simulink model "Pod_elev_plant_mulecola"  (R2022b)
settings: Solver=VariableStepAuto  StartTime=0.0  StopTime=10.0  RelTol=1e-3
undefined symbols (not defined in the file): fix_conseg, fric_gear_elev, JLreg, JMreg, Kkeg, Kveg
settings Model: Creator=ohadformanair  LastModifiedBy=ohadformanair

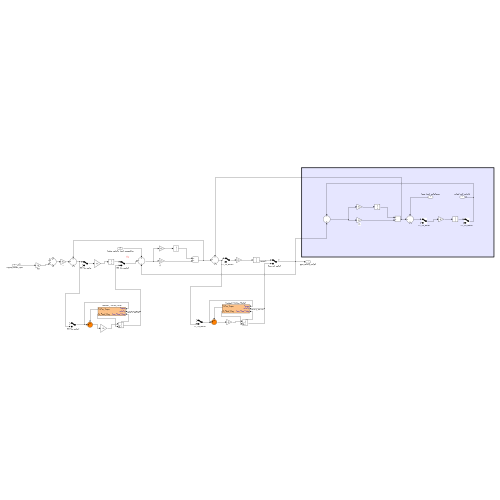
[thumbnail: Simulink's stored preview of the top-level diagram]
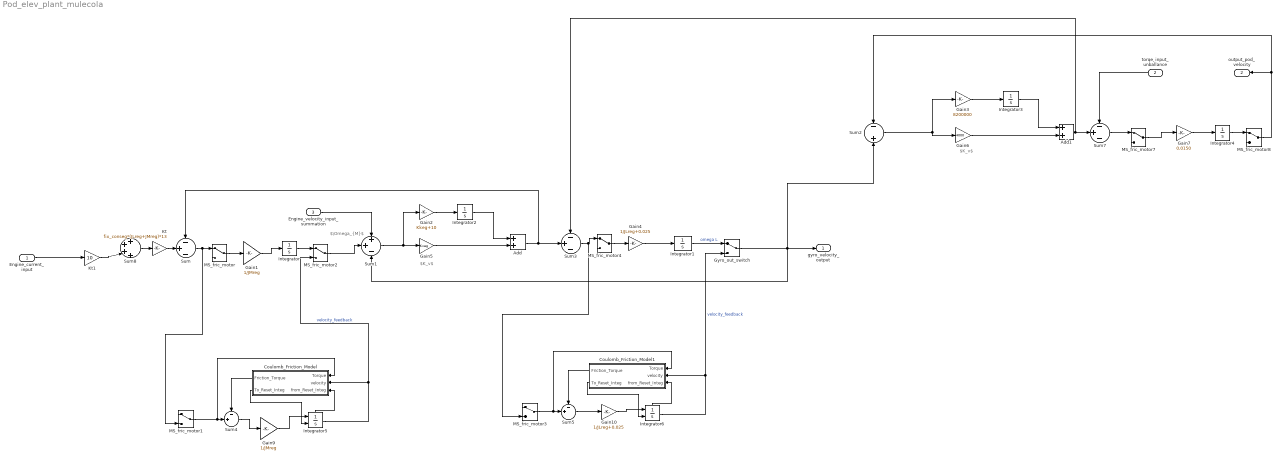
== system Pod_elev_plant_mulecola ==
  note: $K_v$
  note: $K_v$
  note: $\Omega_{M}$
  Engine_current_input : Inport
  torqe_input_unballance : Inport  Port=2
  Engine_velocity_input_summation : Inport  Port=3
  Add : Sum
  Add1 : Sum
  Coulomb_Friction_Model : Subsystem
  Coulomb_Friction_Model1 : Subsystem
  Gain1 : Gain  Gain=1/JMreg
  Gain10 : Gain  Gain=1/JLreg+0.025
  Gain2 : Gain  Gain=Kkeg+10
  Gain3 : Gain  Gain=8200000
  Gain4 : Gain  Gain=1/JLreg+0.025
  Gain5 : Gain  Gain=Kveg
  Gain6 : Gain  Gain=4000
  Gain7 : Gain  Gain=0.0150
  Gain9 : Gain  Gain=1/JMreg
  Gyro_out_switch : ManualSwitch
  Integrator{,1..4} (5 alike) : Integrator
  Integrator5 : Integrator  ExternalReset=rising  ShowStatePort=on
  Integrator6 : Integrator  ExternalReset=rising  ShowStatePort=on
  Kt : Gain  Gain=fix_conseg*(JLreg+JMreg)*13
  Kt1 : Gain  Gain=10
  MS_fric_motor{,1..4,7..8} (7 alike) : ManualSwitch
  Sum : Sum  Inputs=-+-
  Sum1 : Sum  Inputs=++-
  Sum2 : Sum  Inputs=-+
  Sum3 : Sum  Inputs=-+-
  Sum4 : Sum  Inputs=-+|  SaturateOnIntegerOverflow=on
  Sum5 : Sum  Inputs=-+|  SaturateOnIntegerOverflow=on
  Sum7 : Sum  Inputs=-+-
  Sum8 : Sum  Inputs=++++
  gyro_velocity_output : Outport
  output_pod_velocity : Outport  Port=2
  wires:
  Gain1/1 -> Integrator/1
  Sum1/1 -> Gain5/1, Gain2/1
  Integrator2/1 -> Add/1
  Kt1/1 -> Sum8/3
  Gain5/1 -> Add/2
  Gain6/1 -> Add1/2
  Gain7/1 -> Integrator4/1
  Add/1 -> Sum3/2, Sum/1
  Gain3/1 -> Integrator3/1
  Integrator3/1 -> Add1/1
  MS_fric_motor8/1 -> output_pod_velocity/1, Sum2/1
  Gyro_out_switch/1 -> Sum2/2, Sum1/3, gyro_velocity_output/1
  MS_fric_motor2/1 -> Sum1/2
  Integrator4/1 -> MS_fric_motor8/1
  Sum7/1 -> MS_fric_motor7/1
  Gain2/1 -> Integrator2/1
  Sum8/1 -> Kt/1
  MS_fric_motor/1 -> Gain1/1
  Sum2/1 -> Gain6/1, Gain3/1
  Integrator1/1 -> Gyro_out_switch/1  "omega L"
  Engine_current_input/1 -> Kt1/1
  Integrator/1 -> MS_fric_motor2/1
  Sum3/1 -> MS_fric_motor3/2, MS_fric_motor4/1
  Gain4/1 -> Integrator1/1
  MS_fric_motor7/1 -> Gain7/1
  Kt/1 -> Sum/2
  MS_fric_motor4/1 -> Gain4/1
  Sum/1 -> MS_fric_motor1/2, MS_fric_motor/1
  Add1/1 -> Sum7/2, Sum3/1
  torqe_input_unballance/1 -> Sum7/1
  Engine_velocity_input_summation/1 -> Sum1/1
  Gain9/1 -> Integrator5/1
  Integrator5/1 -> MS_fric_motor2/2, Coulomb_Friction_Model/2(velocity)  "velocity_feedback"
  Coulomb_Friction_Model/1(Friction_Torque) -> Sum4/1
  MS_fric_motor1/1 -> Coulomb_Friction_Model/1(Torque), Sum4/2
  Coulomb_Friction_Model/2(To_Reset_Integ) -> Integrator5/2
  Sum4/1 -> Gain9/1
  Integrator5/State -> Coulomb_Friction_Model/3(from_Reset_Integ)
  MS_fric_motor3/1 -> Coulomb_Friction_Model1/1(Torque), Sum5/2
  Gain10/1 -> Integrator6/1
  Coulomb_Friction_Model1/2(To_Reset_Integ) -> Integrator6/2
  Integrator6/1 -> Gyro_out_switch/2, Coulomb_Friction_Model1/2(velocity)  "velocity_feedback"
  Sum5/1 -> Gain10/1
  Integrator6/State -> Coulomb_Friction_Model1/3(from_Reset_Integ)
  Coulomb_Friction_Model1/1(Friction_Torque) -> Sum5/1

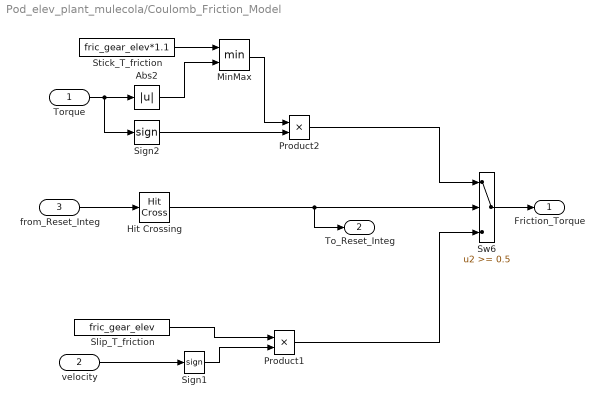
== system Pod_elev_plant_mulecola/Coulomb_Friction_Model ==
  Torque : Inport
  velocity : Inport  Port=2
  from_Reset_Integ : Inport  Port=3
  Abs2 : Abs  SaturateOnIntegerOverflow=off
  Hit Crossing : HitCross  ZeroCross=off
  MinMax : MinMax  Inputs=2
  Product1 : Product  RndMeth=Zero
  Product2 : Product  RndMeth=Zero
  Sign1 : Signum  ZeroCross=off
  Sign2 : Signum  ZeroCross=off
  Slip_T_friction : Constant  Value=fric_gear_elev
  Stick_T_friction : Constant  Value=fric_gear_elev*1.1
  Sw6 : Switch  Threshold=0.5
  Friction_Torque : Outport
  To_Reset_Integ : Outport  Port=2
  wires:
  Torque/1 -> Abs2/1, Sign2/1
  Sw6/1 -> Friction_Torque/1
  velocity/1 -> Sign1/1
  Sign1/1 -> Product1/2
  Product1/1 -> Sw6/3
  Hit Crossing/1 -> To_Reset_Integ/1, Sw6/2
  from_Reset_Integ/1 -> Hit Crossing/1
  Sign2/1 -> Product2/2
  Stick_T_friction/1 -> MinMax/1
  Abs2/1 -> MinMax/2
  MinMax/1 -> Product2/1
  Product2/1 -> Sw6/1
  Slip_T_friction/1 -> Product1/1

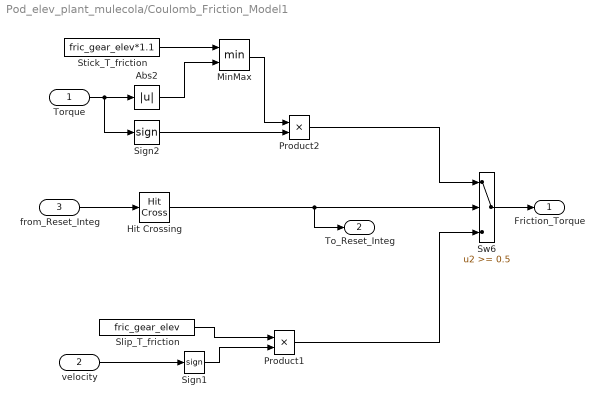
== system Pod_elev_plant_mulecola/Coulomb_Friction_Model1 ==
  Torque : Inport
  velocity : Inport  Port=2
  from_Reset_Integ : Inport  Port=3
  Abs2 : Abs  SaturateOnIntegerOverflow=off
  Hit Crossing : HitCross  ZeroCross=off
  MinMax : MinMax  Inputs=2
  Product1 : Product  RndMeth=Zero
  Product2 : Product  RndMeth=Zero
  Sign1 : Signum  ZeroCross=off
  Sign2 : Signum  ZeroCross=off
  Slip_T_friction : Constant  Value=fric_gear_elev
  Stick_T_friction : Constant  Value=fric_gear_elev*1.1
  Sw6 : Switch  Threshold=0.5
  Friction_Torque : Outport
  To_Reset_Integ : Outport  Port=2
  wires:
  Torque/1 -> Abs2/1, Sign2/1
  Sw6/1 -> Friction_Torque/1
  velocity/1 -> Sign1/1
  Sign1/1 -> Product1/2
  Product1/1 -> Sw6/3
  Hit Crossing/1 -> To_Reset_Integ/1, Sw6/2
  from_Reset_Integ/1 -> Hit Crossing/1
  Sign2/1 -> Product2/2
  Stick_T_friction/1 -> MinMax/1
  Abs2/1 -> MinMax/2
  MinMax/1 -> Product2/1
  Product2/1 -> Sw6/1
  Slip_T_friction/1 -> Product1/1
